simulink model "engine_ol"  (R2018b)
settings: Solver=VariableStepAuto  StartTime=0  StopTime=15  MaxStep=0.01  RelTol=1e-3  EnableMultiTasking=on
model workspace (MAT data in the model file):
  op_engine_ol : opcond.OperatingPoint (value not decoded)
  p = [-7.82997288351e-05; 0.181210895977; -0.072497134344; 0.000486358314052; 0.0361674637937]
settings Model: Creator=The MathWorks Inc.  LastModifiedBy=aturevsk
settings DataIOCC: ExternalInput=getinputstruct(op_engine_ol)  InitialState=getstatestruct(op_engine_ol)  LoadExternalInput=on  LoadInitialState=on  SaveFormat=StructureWithTime  SignalLoggingSaveFormat=ModelDataLogs  SaveOutput=off  SaveTime=off  SignalLoggingName=sigsout
settings OptimizationCC: DefaultParameterBehavior=Inlined  InlineInvariantSignals=on  BufferReuse=off  ExpressionDepthLimit=2147483647  InitFltsAndDblsToZero=on  EfficientMapNaN2IntZero=off  LifeSpan=inf
settings DebuggingCC: SaveWithParameterizedLinksMsg=none  UnderspecifiedInitializationDetection=Classic  MergeDetectMultiDrivingBlocksExec=none  CheckExecutionContextPreStartOutputMsg=on  CheckExecutionContextRuntimeOutputMsg=on  SignalResolutionControl=TryResolveAllWithWarning  SolverPrmCheckMsg=warning  InheritedTsInSrcMsg=none  MultiTaskDSMMsg=warning  FcnCallInpInsideContextMsg=warning  StateNameClashWarn=warning  SFUnexpectedBacktrackingDiag=warning  SFNoUnconditionalDefaultTransitionDiag=warning  SFExecutionAtInitializationDiag=none
settings HardwareCC: ProdBitPerPointer=32  ProdBitPerSizeT=32  ProdBitPerPtrDiffT=32  ProdLargestAtomicFloat=None  ProdIntDivRoundTo=Undefined  ProdEndianess=Unspecified  ProdWordSize=32  ProdHWDeviceType=32-bit Generic
settings ModelReferenceCC: PropagateSignalLabelsOutOfModel=off
settings SFSimCC: SimUseLocalCustomCode=off
settings RTWCC: RTWUseLocalCustomCode=off
settings CodeAppCC: StateflowObjectComments=on
settings GRTTargetCC: TargetFcnLib=ansi_tfl_tmw.mat  TargetLangStandard=C89/C90 (ANSI)  GeneratePreprocessorConditionals=Disable all  CombineOutputUpdateFcns=off  GRTInterface=on
settings ConfigComp: CovMetricSettings=dw  CovHtmlReporting=on  CovSaveCumulativeToWorkspaceVar=on  CovSaveSingleToWorkspaceVar=on  CovExternalEMLEnable=off

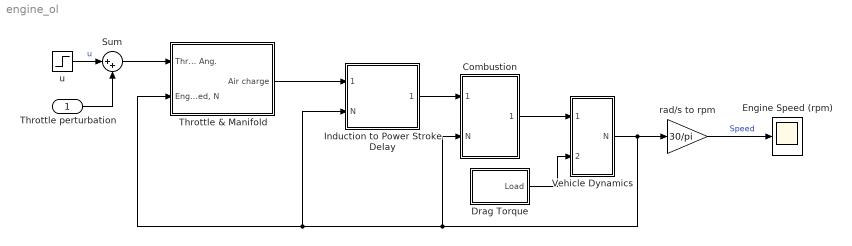
== system engine_ol ==
  Throttle perturbation : Inport
  Combustion : Subsystem
      settings: RTWMemSecFuncInitTerm=Default  RTWMemSecFuncExecute=Default  RTWMemSecDataConstants=Default  RTWMemSecDataInternal=Default  RTWMemSecDataParameters=Default
  Drag Torque : Subsystem
      settings: RTWMemSecFuncInitTerm=Default  RTWMemSecFuncExecute=Default  RTWMemSecDataConstants=Default  RTWMemSecDataInternal=Default  RTWMemSecDataParameters=Default
  Engine Speed (rpm) : Scope
  Induction to Power Stroke Delay : Subsystem
      settings: RTWMemSecFuncInitTerm=Default  RTWMemSecFuncExecute=Default  RTWMemSecDataConstants=Default  RTWMemSecDataInternal=Default  RTWMemSecDataParameters=Default
  Sum : Sum  Inputs=|++
  Throttle & Manifold : Subsystem
      settings: RTWMemSecFuncInitTerm=Default  RTWMemSecFuncExecute=Default  RTWMemSecDataConstants=Default  RTWMemSecDataInternal=Default  RTWMemSecDataParameters=Default
  Vehicle Dynamics : Subsystem
      settings: RTWMemSecFuncInitTerm=Default  RTWMemSecFuncExecute=Default  RTWMemSecDataConstants=Default  RTWMemSecDataInternal=Default  RTWMemSecDataParameters=Default
  rad/s to rpm : Gain  Gain=30/pi  SaturateOnIntegerOverflow=on  OutDataTypeStr=Inherit: Same as input  ParamDataTypeStr=Inherit: Same as input
  u : Step  Time=2  Before=9  After=9.5
  wires:
  Throttle & Manifold/1(Air charge) -> Induction to Power Stroke Delay/1(Air charge)
  Vehicle Dynamics/1(N) -> Combustion/2(N), Induction to Power Stroke Delay/2(N), Throttle & Manifold/2("Engine Speed, N"), rad/s to rpm/1
  Combustion/1(Torque) -> Vehicle Dynamics/1(Teng)
  Drag Torque/1(Load) -> Vehicle Dynamics/2(Tload)
  Induction to Power Stroke Delay/1(Air Charge) -> Combustion/1(Air Charge)
  rad/s to rpm/1 -> Engine Speed (rpm)/1  "Speed"
  u/1 -> Sum/1  "u"
  Throttle perturbation/1 -> Sum/2
  Sum/1 -> Throttle & Manifold/1(Throttle Ang.)

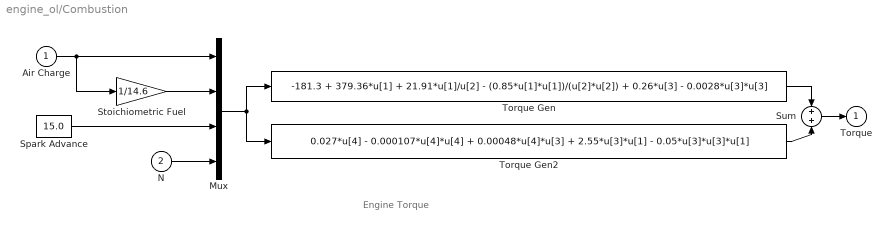
== system engine_ol/Combustion ==
  note: Engine Torque
  Air Charge : Inport
  N : Inport  Port=2
  Mux : Mux
  Spark Advance : Constant  Value=15.0
  Stoichiometric Fuel : Gain  Gain=1/14.6  SaturateOnIntegerOverflow=on  OutDataTypeStr=Inherit: Same as input  ParamDataTypeStr=Inherit: Same as input
  Sum : Sum  SaturateOnIntegerOverflow=on  InputSameDT=on  OutDataTypeStr=Inherit: Same as first input
  Torque Gen : Fcn  Expr=-181.3 + 379.36*u[1] + 21.91*u[1]/u[2] - (0.85*u[1]*u[1])/(u[2]*u[2]) + 0.26*u[3] - 0.0028*u[3]*u[3]
  Torque Gen2 : Fcn  Expr=0.027*u[4] - 0.000107*u[4]*u[4] + 0.00048*u[4]*u[3] + 2.55*u[3]*u[1] - 0.05*u[3]*u[3]*u[1]
  Torque : Outport  InitialOutput=0
  wires:
  Stoichiometric Fuel/1 -> Mux/2
  Spark Advance/1 -> Mux/3
  N/1 -> Mux/4
  Air Charge/1 -> Stoichiometric Fuel/1, Mux/1
  Mux/1 -> Torque Gen/1, Torque Gen2/1
  Torque Gen2/1 -> Sum/2
  Torque Gen/1 -> Sum/1
  Sum/1 -> Torque/1

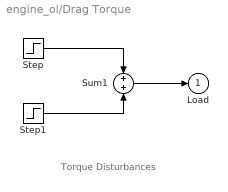
== system engine_ol/Drag Torque ==
  note: Torque Disturbances
  Step : Step  Time=2  Before=25  After=25  SampleTime=0
  Step1 : Step  Time=8  After=0  SampleTime=0
  Sum1 : Sum  SaturateOnIntegerOverflow=on  InputSameDT=on  OutDataTypeStr=Inherit: Same as first input
  Load : Outport  InitialOutput=0
  wires:
  Step1/1 -> Sum1/2
  Step/1 -> Sum1/1
  Sum1/1 -> Load/1

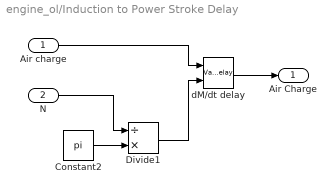
== system engine_ol/Induction to Power Stroke Delay ==
  Air charge : Inport
  N : Inport  Port=2
  Constant2 : Constant  Value=pi
  Divide1 : Product  Inputs=/*
  dM/dt delay : VariableTransportDelay  MaximumDelay=10  InitialOutput=0.152  MaximumPoints=10240  TransDelayFeedthrough=on  PadeOrder=2
  Air Charge : Outport
  wires:
  dM/dt delay/1 -> Air Charge/1
  Constant2/1 -> Divide1/2
  N/1 -> Divide1/1
  Divide1/1 -> dM/dt delay/2
  Air charge/1 -> dM/dt delay/1

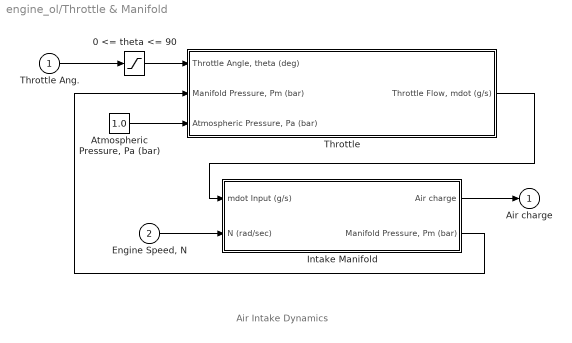
== system engine_ol/Throttle & Manifold ==
  note: Air Intake Dynamics
  Throttle Ang. : Inport
  "Engine Speed, N" : Inport  Port=2
  0 <= theta <= 90 : Saturate  UpperLimit=90  LowerLimit=0
  "Atmospheric Pressure, Pa (bar)" : Constant  Value=1.0
  Intake Manifold : Subsystem
      settings: RTWMemSecFuncInitTerm=Default  RTWMemSecFuncExecute=Default  RTWMemSecDataConstants=Default  RTWMemSecDataInternal=Default  RTWMemSecDataParameters=Default
  Throttle : Subsystem
      settings: RTWMemSecFuncInitTerm=Default  RTWMemSecFuncExecute=Default  RTWMemSecDataConstants=Default  RTWMemSecDataInternal=Default  RTWMemSecDataParameters=Default
  Air charge : Outport  InitialOutput=0
  wires:
  "Atmospheric Pressure, Pa (bar)"/1 -> Throttle/3("Atmospheric Pressure, Pa (bar) ")
  Intake Manifold/1(Air charge) -> Air charge/1
  Intake Manifold/2("Manifold Pressure, Pm (bar)") -> Throttle/2("Manifold Pressure, Pm (bar)")
  "Engine Speed, N"/1 -> Intake Manifold/2(N (rad/sec))
  Throttle/1("Throttle Flow, mdot (g/s)") -> Intake Manifold/1(mdot Input (g/s))
  Throttle Ang./1 -> 0 <= theta <= 90/1
  0 <= theta <= 90/1 -> Throttle/1("Throttle Angle, theta (deg)")

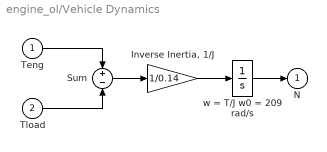
== system engine_ol/Vehicle Dynamics ==
  Teng : Inport
  Tload : Inport  Port=2
  "Inverse Inertia, 1/J" : Gain  Gain=1/0.14  SaturateOnIntegerOverflow=on  OutDataTypeStr=Inherit: Same as input  ParamDataTypeStr=Inherit: Same as input
  Sum : Sum  Inputs=+-  SaturateOnIntegerOverflow=on  InputSameDT=on  OutDataTypeStr=Inherit: Same as first input
  w = T/J w0 = 209 rad/s : Integrator  InitialCondition=209.48
  N : Outport  InitialOutput=0
  wires:
  "Inverse Inertia, 1/J"/1 -> w = T/J w0 = 209 rad/s/1
  w = T/J w0 = 209 rad/s/1 -> N/1
  Sum/1 -> "Inverse Inertia, 1/J"/1
  Teng/1 -> Sum/1
  Tload/1 -> Sum/2

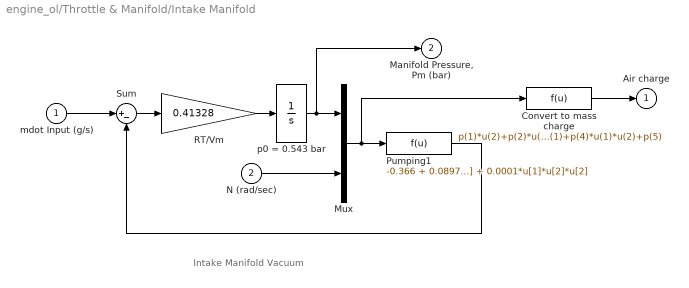
== system engine_ol/Throttle & Manifold/Intake Manifold ==
  note: Intake Manifold Vacuum
  mdot Input (g/s) : Inport
  N (rad/sec) : Inport  Port=2
  Convert to mass charge : Fcn  Expr=p(1)*u(2)+p(2)*u(1)+p(3)*u(1)*u(1)+p(4)*u(1)*u(2)+p(5)
  Mux : Mux  Inputs=2
  Pumping1 : Fcn  Expr=-0.366 + 0.08979*u[1]*u[2] - 0.0337*u[2]*u[1]*u[1] + 0.0001*u[1]*u[2]*u[2]
  RT/Vm : Gain  Gain=0.41328  SaturateOnIntegerOverflow=on  OutDataTypeStr=Inherit: Same as input  ParamDataTypeStr=Inherit: Same as input
  Sum : Sum  Inputs=|+-  SaturateOnIntegerOverflow=on  InputSameDT=on  OutDataTypeStr=Inherit: Same as first input
  p0 = 0.543 bar : Integrator  InitialCondition=.543
  Air charge : Outport  InitialOutput=0
  "Manifold Pressure, Pm (bar)" : Outport  Port=2  InitialOutput=0
  wires:
  Pumping1/1 -> Sum/2
  Sum/1 -> RT/Vm/1
  p0 = 0.543 bar/1 -> "Manifold Pressure, Pm (bar)"/1, Mux/1
  Mux/1 -> Pumping1/1, Convert to mass charge/1
  N (rad/sec)/1 -> Mux/2
  RT/Vm/1 -> p0 = 0.543 bar/1
  mdot Input (g/s)/1 -> Sum/1
  Convert to mass charge/1 -> Air charge/1

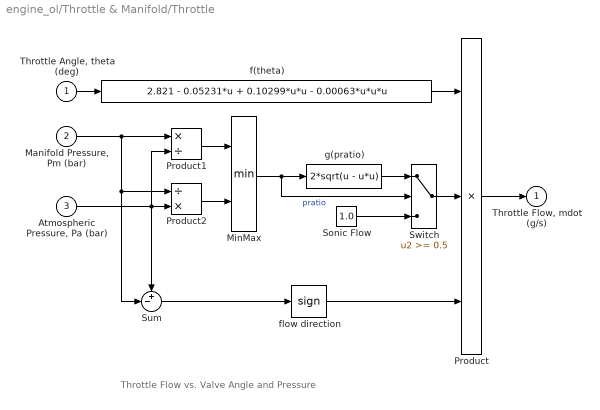
== system engine_ol/Throttle & Manifold/Throttle ==
  note: Throttle Flow vs. Valve Angle and Pressure
  "Throttle Angle, theta (deg)" : Inport
  "Manifold Pressure, Pm (bar)" : Inport  Port=2
  "Atmospheric Pressure, Pa (bar) " : Inport  Port=3
  MinMax : MinMax  Inputs=2  SaturateOnIntegerOverflow=on  InputSameDT=on
  Product : Product  Inputs=3  SaturateOnIntegerOverflow=on  RndMeth=Zero  InputSameDT=on  OutDataTypeStr=Inherit: Same as first input
  Product1 : Product  Inputs=*/  SaturateOnIntegerOverflow=on  RndMeth=Zero  InputSameDT=on  OutDataTypeStr=Inherit: Same as first input
  Product2 : Product  Inputs=/*  SaturateOnIntegerOverflow=on  RndMeth=Zero  InputSameDT=on  OutDataTypeStr=Inherit: Same as first input
  "Sonic Flow " : Constant  Value=1.0
  Sum : Sum  Inputs=+-|  SaturateOnIntegerOverflow=on  InputSameDT=on  OutDataTypeStr=Inherit: Same as first input
  Switch : Switch  Threshold=0.5  SaturateOnIntegerOverflow=on  InputSameDT=on
  f(theta) : Fcn  Expr=2.821 - 0.05231*u + 0.10299*u*u - 0.00063*u*u*u
  flow direction : Signum
  g(pratio) : Fcn  Expr=2*sqrt(u - u*u)
  "Throttle Flow, mdot (g/s)" : Outport  InitialOutput=0
  wires:
  f(theta)/1 -> Product/1
  Product/1 -> "Throttle Flow, mdot (g/s)"/1
  "Throttle Angle, theta (deg)"/1 -> f(theta)/1
  MinMax/1 -> g(pratio)/1, Switch/2  "pratio"
  Sum/1 -> flow direction/1
  flow direction/1 -> Product/3
  Switch/1 -> Product/2
  "Sonic Flow "/1 -> Switch/3
  g(pratio)/1 -> Switch/1
  "Atmospheric Pressure, Pa (bar) "/1 -> Product1/2, Product2/2, Sum/1
  Product1/1 -> MinMax/1
  Product2/1 -> MinMax/2
  "Manifold Pressure, Pm (bar)"/1 -> Product1/1, Product2/1, Sum/2
